simulink model "sampleModel1944_3_sub_sub_sub"  (R2023a)
settings: Solver=VariableStepAuto  StartTime=0.0  StopTime=10.0  RelTol=1e-3
libraries: hdlsllib x6, simulink x1
settings Model: Creator=user1  LastModifiedBy=user1

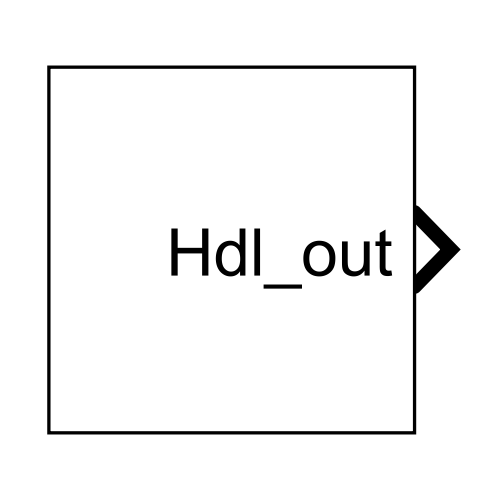
[thumbnail: Simulink's stored preview of the top-level diagram]
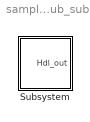
== system sampleModel1944_3_sub_sub_sub ==
  Subsystem : Subsystem

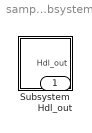
== system sampleModel1944_3_sub_sub_sub/Subsystem ==
  Subsystem : Subsystem
  Hdl_out : Outport  OutDataTypeStr=uint8

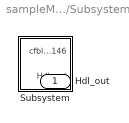
== system sampleModel1944_3_sub_sub_sub/Subsystem/Subsystem ==
  Subsystem : Subsystem
  Hdl_out : Outport  OutDataTypeStr=uint8

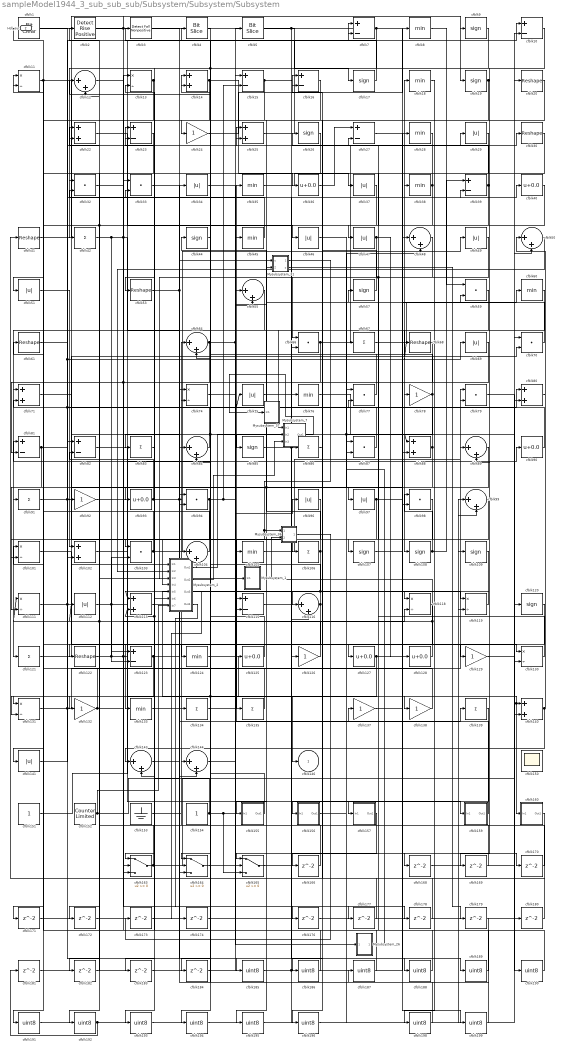
== system sampleModel1944_3_sub_sub_sub/Subsystem/Subsystem/Subsystem ==
  Mysubsystem_1 : Subsystem  TreatAsAtomicUnit=on  RTWFcnName=Mysubsystem_1
      settings: RTWFcnNameOpts=User specified  RTWFileNameOpts=Use function name
  Mysubsystem_2 : Subsystem  TreatAsAtomicUnit=on  RTWFcnName=Mysubsystem_2
      settings: RTWFcnNameOpts=User specified  RTWFileNameOpts=Use function name
  Mysubsystem_26 : Subsystem  TreatAsAtomicUnit=on  RTWFcnName=Mysubsystem_26
      settings: RTWFcnNameOpts=User specified  RTWFileNameOpts=Use function name
  Mysubsystem_31 : Subsystem  TreatAsAtomicUnit=on  RTWFcnName=Mysubsystem_31
      settings: RTWFcnNameOpts=User specified  RTWFileNameOpts=Use function name
  Mysubsystem_36 : Subsystem  TreatAsAtomicUnit=on  RTWFcnName=Mysubsystem_36
      settings: RTWFcnNameOpts=User specified  RTWFileNameOpts=Use function name
  Mysubsystem_37 : Subsystem  TreatAsAtomicUnit=on  RTWFcnName=Mysubsystem_37
      settings: RTWFcnNameOpts=User specified  RTWFileNameOpts=Use function name
  Mysubsystem_7 : Subsystem  TreatAsAtomicUnit=on  RTWFcnName=Mysubsystem_7
      settings: RTWFcnNameOpts=User specified  RTWFileNameOpts=Use function name
  cfblk1 : simulink/Logic and Bit Operations/Bit Clear  iBit=0
      settings: LibrarySourceBlock=|
      | hdlsllib/Logic and Bit
      | Operations/Bit Clear
  cfblk{7,10,15..16,23,27,39,81..82,115,123} (11 alike) : Sum  Inputs=+-  OutDataTypeStr=uint8
  cfblk{11,13,74,101,111,118..119,130..131} (9 alike) : Product  Inputs=*/  OutDataTypeStr=uint8  RndMeth=Zero  SaturateOnIntegerOverflow=on
  cfblk{14,22,25,71,80,88,102,113,140} (9 alike) : Sum  OutDataTypeStr=uint8
  cfblk{32..33,59,66,70,77,79,87,94,98,103} (11 alike) : DotProduct  OutDataTypeStr=uint8
  cfblk{12,48,50,55,64,84,89,99,104,116,143..144} (12 alike) : Sum  Inputs=|++  OutDataTypeStr=uint8
  cfblk{8,18,28,35,38,45,60,76,105,124,133} (11 alike) : MinMax  OutDataTypeStr=uint8
  cfblk{42,67,83,86,91,106,121,134..135,139} (10 alike) : Sum  Inputs=+  OutDataTypeStr=uint8
  cfblk{9,17,19,26,44,57,85,107..109,120} (11 alike) : Signum
  cfblk{29,34,37,46..47,49,51,69,75,96..97,112,141} (13 alike) : Abs  OutDataTypeStr=uint8  SaturateOnIntegerOverflow=off
  cfblk{20,30,41,53,61,68,122} (7 alike) : Reshape
  cfblk{36,40,90,93,125,127..128} (7 alike) : Bias  Bias=0.0  SaturateOnIntegerOverflow=off
  cfblk{24,78,92,126,129,132,137..138} (8 alike) : Gain  OutDataTypeStr=uint8
  cfblk150 : Scope
      settings: Floating=on
  cfblk151 : Constant  OutDataTypeStr=uint8  SampleTime=-1
  cfblk152 : hdlsllib/Sources/Counter Limited  uplimit=7  tsamp=-1
  cfblk153 : Ground
  cfblk154 : Constant  OutDataTypeStr=uint8  SampleTime=-1
  cfblk155 : Subsystem
      settings: LibrarySourceBlock=|
      | hdlsllib/Ports &
      | Subsystems/Subsystem
  cfblk156 : Subsystem
      settings: LibrarySourceBlock=|
      | hdlsllib/Ports &
      | Subsystems/Subsystem
  cfblk157 : Subsystem
      settings: LibrarySourceBlock=|
      | hdlsllib/Ports &
      | Subsystems/Subsystem
  cfblk159 : Subsystem
      settings: LibrarySourceBlock=|
      | hdlsllib/Ports &
      | Subsystems/Subsystem
  cfblk160 : Subsystem
      settings: LibrarySourceBlock=|
      | hdlsllib/Ports &
      | Subsystems/Subsystem
  cfblk163 : Switch  OutDataTypeStr=uint8  SaturateOnIntegerOverflow=off  InputSameDT=off
  cfblk164 : Switch  OutDataTypeStr=uint8  SaturateOnIntegerOverflow=off  InputSameDT=off
  cfblk165 : Switch  OutDataTypeStr=uint8  SaturateOnIntegerOverflow=off  InputSameDT=off
  cfblk{166,168..174,176..184} (17 alike) : Delay  SampleTime=1
  cfblk{185..196,198..199} (14 alike) : DataTypeConversion  OutDataTypeStr=uint8  SaturateOnIntegerOverflow=off  RndMeth=Floor
  cfblk2 : hdlsllib/Logic and Bit Operations/Detect Rise Positive  vinit=0  OutDataTypeStr=uint8
  cfblk3 : hdlsllib/Logic and Bit Operations/Detect Fall Nonpositive  vinit=0  OutDataTypeStr=uint8
  cfblk4 : hdlsllib/Logic and Bit Operations/Bit Slice  lidx=7  ridx=0
  cfblk5 : hdlsllib/Logic and Bit Operations/Bit Slice  lidx=7  ridx=0
  cfblk146 : Outport  OutDataTypeStr=uint8  VectorParamsAs1DForOutWhenUnconnected=off
  Hdl_out : Outport  Port=2  OutDataTypeStr=uint8
  wires:
  cfblk22/1 -> cfblk46/1
  cfblk8/1 -> cfblk59/1
  cfblk80/1 -> cfblk121/1
  cfblk159/1(Out1) -> cfblk35/1
  cfblk66/1 -> cfblk164/2, cfblk29/1
  cfblk36/1 -> cfblk27/1
  cfblk93/1 -> cfblk12/2, cfblk177/1, cfblk49/1
  cfblk157/1(Out1) -> cfblk165/1
  cfblk121/1 -> cfblk70/2
  cfblk41/1 -> cfblk19/1
  cfblk153/1 -> cfblk64/1
  cfblk51/1 -> cfblk102/1
  cfblk91/1 -> cfblk25/1, cfblk97/1
  cfblk5/1 -> cfblk188/1, cfblk17/1
  cfblk160/1(Out1) -> cfblk41/1
  cfblk25/1 -> cfblk7/1
  cfblk101/1 -> cfblk127/1
  cfblk119/1 -> cfblk116/1
  cfblk57/1 -> cfblk16/1
  cfblk151/1 -> cfblk10/1
  cfblk15/1 -> cfblk130/2, cfblk124/1
  cfblk16/1 -> cfblk85/1
  cfblk37/1 -> cfblk122/1
  cfblk17/1 -> cfblk3/1
  cfblk88/1 -> cfblk27/2, cfblk115/1, cfblk131/1
  cfblk60/1 -> cfblk108/1
  cfblk35/1 -> cfblk37/1
  cfblk123/1 -> cfblk104/2, cfblk131/2
  cfblk131/1 -> cfblk79/1, cfblk75/1, cfblk25/2, cfblk68/1
  cfblk112/1 -> cfblk123/2, cfblk157/1(In1)
  cfblk48/1 -> cfblk107/1, Mysubsystem_2/3(In3)
  cfblk40/1 -> cfblk155/1(In1)
  cfblk64/1 -> cfblk138/1, cfblk5/1, cfblk81/2, cfblk163/2
  cfblk107/1 -> cfblk80/1
  cfblk103/1 -> cfblk11/2, cfblk18/1
  cfblk120/1 -> cfblk133/1
  cfblk77/1 -> cfblk45/1
  cfblk87/1 -> cfblk23/1
  cfblk138/1 -> cfblk101/1
  cfblk105/1 -> cfblk89/1
  cfblk122/1 -> cfblk103/2, cfblk39/2, cfblk79/2
  cfblk128/1 -> cfblk111/1, Mysubsystem_36/2(In2)
  cfblk89/1 -> cfblk172/1, Mysubsystem_31/2(In2)
  cfblk33/1 -> cfblk185/1
  cfblk90/1 -> cfblk14/1
  cfblk81/1 -> cfblk40/1, cfblk101/2
  cfblk140/1 -> cfblk50/1, cfblk143/1
  cfblk20/1 -> cfblk24/1
  cfblk11/1 -> cfblk51/1, cfblk135/1
  cfblk53/1 -> cfblk119/1, Mysubsystem_31/1(u)
  cfblk144/1 -> cfblk137/1
  cfblk135/1 -> cfblk14/2
  cfblk82/1 -> cfblk146/1
  cfblk92/1 -> cfblk20/1
  cfblk111/1 -> cfblk7/2, cfblk34/1
  cfblk30/1 -> cfblk47/1
  cfblk130/1 -> cfblk57/1
  cfblk137/1 -> cfblk28/1
  cfblk124/1 -> cfblk140/1, cfblk160/1(In1)
  cfblk127/1 -> cfblk140/2, cfblk194/1, Mysubsystem_2/5(In5)
  cfblk94/1 -> cfblk102/2, cfblk15/2, cfblk15/1
  cfblk55/1 -> cfblk132/1
  cfblk9/1 -> cfblk42/1
  cfblk34/1 -> cfblk159/1(In1)
  cfblk106/1 -> cfblk164/3, cfblk55/1
  cfblk70/1 -> cfblk44/1
  cfblk141/1 -> cfblk82/1
  cfblk44/1 -> cfblk64/2
  cfblk125/1 -> cfblk81/1
  cfblk102/1 -> cfblk90/1
  cfblk42/1 -> cfblk123/1, cfblk125/1, cfblk104/1
  cfblk116/1 -> cfblk171/1, cfblk32/2, cfblk113/1
  cfblk69/1 -> cfblk93/1
  cfblk71/1 -> cfblk144/2
  cfblk3/1 -> cfblk94/1
  cfblk13/1 -> cfblk141/1, cfblk83/1
  cfblk7/1 -> Hdl_out/1, cfblk199/1, cfblk164/1, cfblk53/1
  cfblk83/1 -> cfblk143/2
  cfblk156/1(Out1) -> cfblk48/2
  cfblk133/1 -> cfblk84/1
  cfblk143/1 -> cfblk139/1
  cfblk104/1 -> cfblk22/1
  cfblk28/1 -> cfblk86/1
  cfblk134/1 -> cfblk55/2
  cfblk4/1 -> cfblk84/2
  cfblk2/1 -> cfblk9/1, cfblk106/1
  cfblk108/1 -> cfblk39/1, cfblk98/1
  cfblk97/1 -> cfblk111/2, cfblk59/2
  cfblk45/1 -> cfblk13/2
  cfblk23/1 -> cfblk71/1
  cfblk24/1 -> cfblk8/1
  cfblk86/1 -> cfblk156/1(In1)
  cfblk129/1 -> cfblk10/2
  cfblk29/1 -> cfblk105/1
  cfblk132/1 -> cfblk118/2, cfblk61/1
  cfblk26/1 -> cfblk92/1
  cfblk113/1 -> cfblk69/1
  cfblk39/1 -> cfblk198/1, cfblk26/1
  cfblk27/1 -> cfblk129/1
  cfblk67/1 -> cfblk60/1
  cfblk154/1 -> cfblk113/2, Mysubsystem_2/6(In6), cfblk165/3, cfblk96/1
  cfblk164/1 -> cfblk165/2
  cfblk79/1 -> cfblk120/1
  cfblk96/1 -> cfblk103/1
  cfblk85/1 -> cfblk38/1, cfblk118/1
  cfblk155/1(Out1) -> cfblk12/1
  cfblk163/1 -> cfblk50/2, cfblk82/2
  cfblk126/1 -> cfblk112/1, Mysubsystem_1/1(In1)
  cfblk14/1 -> cfblk163/3, cfblk36/1
  cfblk98/1 -> cfblk163/1
  cfblk19/1 -> cfblk186/1, cfblk89/2
  cfblk47/1 -> cfblk196/1, cfblk128/1
  cfblk115/1 -> cfblk130/1
  cfblk99/1 -> cfblk192/1
  cfblk84/1 -> cfblk11/1
  cfblk49/1 -> cfblk66/1
  cfblk78/1 -> cfblk4/1, cfblk184/1, cfblk183/1
  cfblk38/1 -> cfblk32/1, cfblk182/1, cfblk91/1
  cfblk61/1 -> cfblk30/1
  cfblk152/1 -> cfblk134/1, Mysubsystem_2/7(In7)
  cfblk46/1 -> cfblk88/1, cfblk98/2
  cfblk18/1 -> cfblk78/1
  cfblk139/1 -> cfblk166/1
  cfblk166/1 -> cfblk13/1
  cfblk165/1 -> cfblk168/1
  cfblk168/1 -> cfblk70/1
  cfblk10/1 -> cfblk169/1
  cfblk169/1 -> cfblk144/1
  cfblk75/1 -> cfblk170/1
  cfblk170/1 -> cfblk2/1
  cfblk171/1 -> cfblk119/2
  cfblk172/1 -> cfblk116/2
  cfblk173/1 -> cfblk80/2
  cfblk174/1 -> cfblk66/2
  cfblk176/1 -> cfblk48/1
  cfblk177/1 -> cfblk71/2
  cfblk32/1 -> cfblk178/1
  cfblk178/1 -> cfblk23/2
  cfblk180/1 -> cfblk16/2
  cfblk181/1 -> cfblk94/2
  cfblk182/1 -> cfblk22/2
  cfblk183/1 -> cfblk115/2
  cfblk184/1 -> cfblk88/2
  cfblk185/1 -> cfblk67/1, cfblk126/1
  cfblk186/1 -> cfblk33/1
  cfblk179/1 -> cfblk187/1
  cfblk187/1 -> cfblk33/2
  cfblk188/1 -> cfblk1/1
  cfblk1/1 -> cfblk189/1
  cfblk189/1 -> cfblk77/1
  cfblk76/1 -> cfblk190/1
  cfblk190/1 -> cfblk77/2
  cfblk68/1 -> cfblk191/1
  cfblk191/1 -> cfblk76/1
  cfblk192/1 -> cfblk180/1, cfblk181/1
  cfblk118/1 -> cfblk193/1
  cfblk193/1 -> cfblk99/1
  cfblk194/1 -> cfblk99/2
  cfblk109/1 -> cfblk195/1
  cfblk195/1 -> cfblk87/2
  cfblk196/1 -> cfblk109/1
  cfblk198/1 -> cfblk74/1
  cfblk199/1 -> cfblk74/2
  cfblk12/1 -> Mysubsystem_2/1(In1)
  cfblk50/1 -> Mysubsystem_2/2(In2)
  Mysubsystem_2/3(Out3) -> cfblk174/1
  Mysubsystem_2/4(Out4) -> cfblk176/1
  cfblk59/1 -> Mysubsystem_7/1(In1)
  Mysubsystem_2/1(Out1) -> Mysubsystem_7/2(In2)
  Mysubsystem_2/2(Out2) -> Mysubsystem_7/3(In3)
  cfblk74/1 -> Mysubsystem_26/1(In1)
  Mysubsystem_26/1(Out1) -> cfblk87/1
  Mysubsystem_31/1(Out1) -> Mysubsystem_2/4(In4), Mysubsystem_36/1(In1)
  Mysubsystem_31/2(y) -> cfblk179/1
  Mysubsystem_36/1(Out1) -> cfblk173/1
  Mysubsystem_7/1(Out1) -> Mysubsystem_37/1(In1)

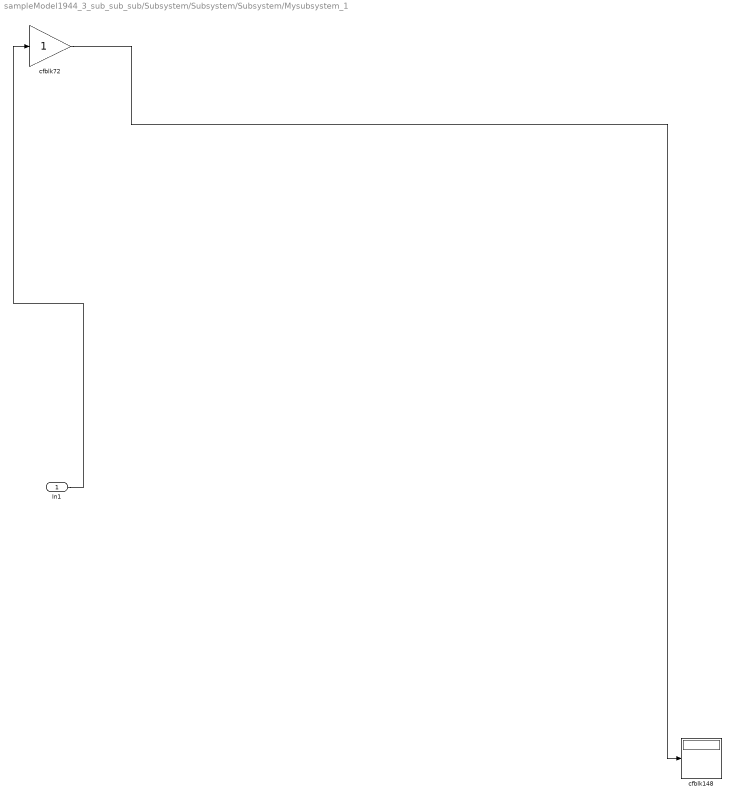
== system sampleModel1944_3_sub_sub_sub/Subsystem/Subsystem/Subsystem/Mysubsystem_1 ==
  In1 : Inport
  cfblk148 : Display
  cfblk72 : Gain
  wires:
  In1/1 -> cfblk72/1
  cfblk72/1 -> cfblk148/1

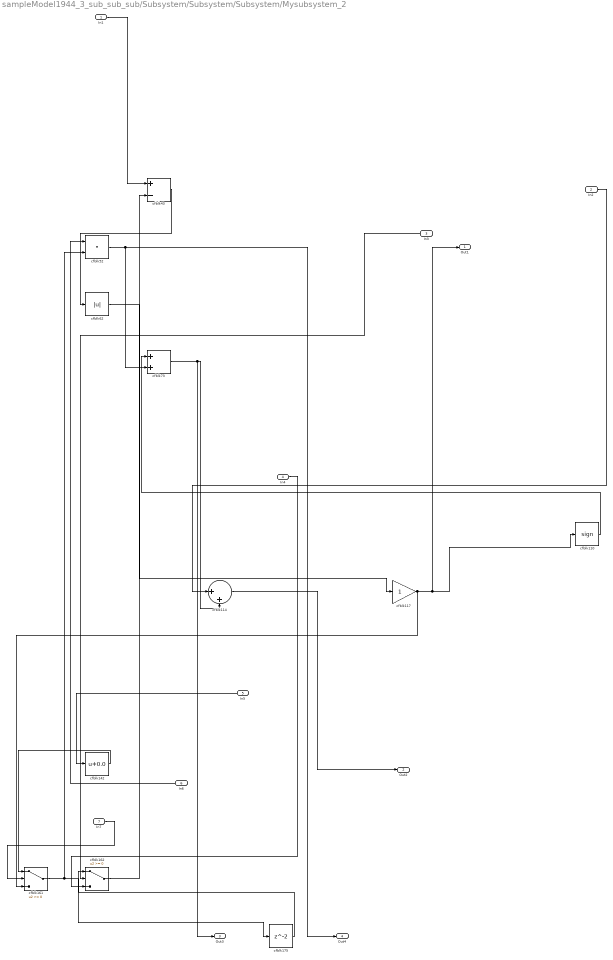
== system sampleModel1944_3_sub_sub_sub/Subsystem/Subsystem/Subsystem/Mysubsystem_2 ==
  In1 : Inport
  In2 : Inport  Port=2
  In3 : Inport  Port=3
  In4 : Inport  Port=4
  In5 : Inport  Port=5
  In6 : Inport  Port=6
  In7 : Inport  Port=7
  cfblk110 : Signum
  cfblk114 : Sum  Inputs=|++
  cfblk117 : Gain
  cfblk142 : Bias  Bias=0.0  SaturateOnIntegerOverflow=off
  cfblk161 : Switch  SaturateOnIntegerOverflow=off  InputSameDT=off
  cfblk162 : Switch  SaturateOnIntegerOverflow=off  InputSameDT=off
  cfblk175 : Delay  SampleTime=1
  cfblk43 : Sum  Inputs=+-
  cfblk52 : DotProduct  OutDataTypeStr=Inherit: Inherit via internal rule
  cfblk62 : Abs  SaturateOnIntegerOverflow=off
  cfblk73 : Sum
  Out1 : Outport
  Out2 : Outport  Port=2
  Out3 : Outport  Port=3
  Out4 : Outport  Port=4
  wires:
  In3/1 -> cfblk162/2
  In6/1 -> cfblk52/1
  In5/1 -> cfblk142/1
  In2/1 -> cfblk114/1
  cfblk114/1 -> Out2/1
  cfblk175/1 -> cfblk162/1
  cfblk162/1 -> cfblk43/2
  In4/1 -> cfblk162/3
  cfblk43/1 -> cfblk62/1
  cfblk52/1 -> cfblk73/2, Out4/1
  cfblk62/1 -> cfblk117/1
  cfblk117/1 -> cfblk161/3, cfblk110/1, Out1/1
  In1/1 -> cfblk43/1
  In7/1 -> cfblk161/2
  cfblk110/1 -> cfblk73/1
  cfblk142/1 -> cfblk161/1
  cfblk161/1 -> cfblk175/1, cfblk52/2
  cfblk73/1 -> cfblk114/2, Out3/1

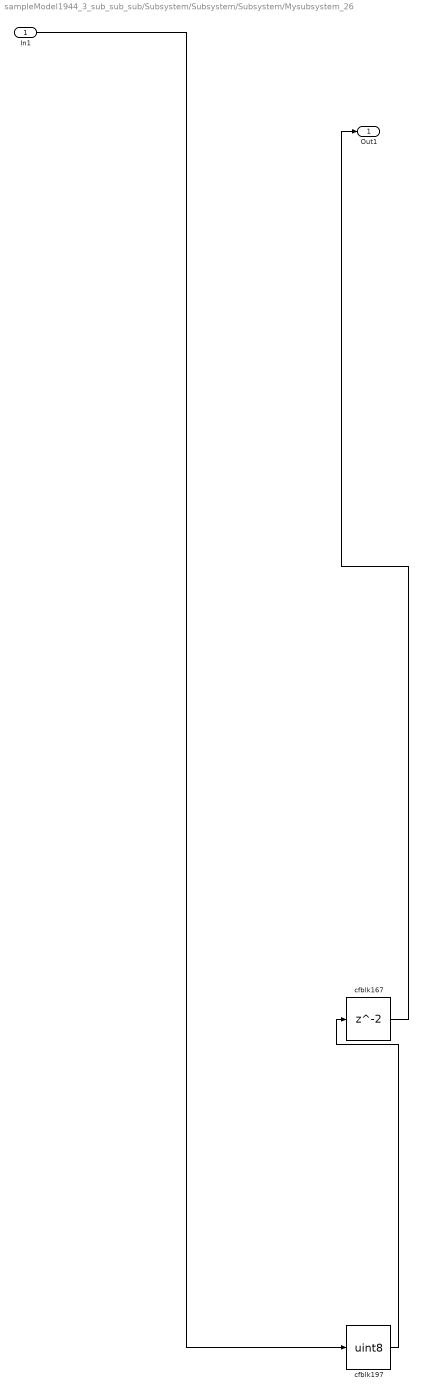
== system sampleModel1944_3_sub_sub_sub/Subsystem/Subsystem/Subsystem/Mysubsystem_26 ==
  In1 : Inport
  cfblk167 : Delay  SampleTime=1
  cfblk197 : DataTypeConversion  OutDataTypeStr=uint8  SaturateOnIntegerOverflow=off  RndMeth=Floor
  Out1 : Outport
  wires:
  In1/1 -> cfblk197/1
  cfblk167/1 -> Out1/1
  cfblk197/1 -> cfblk167/1

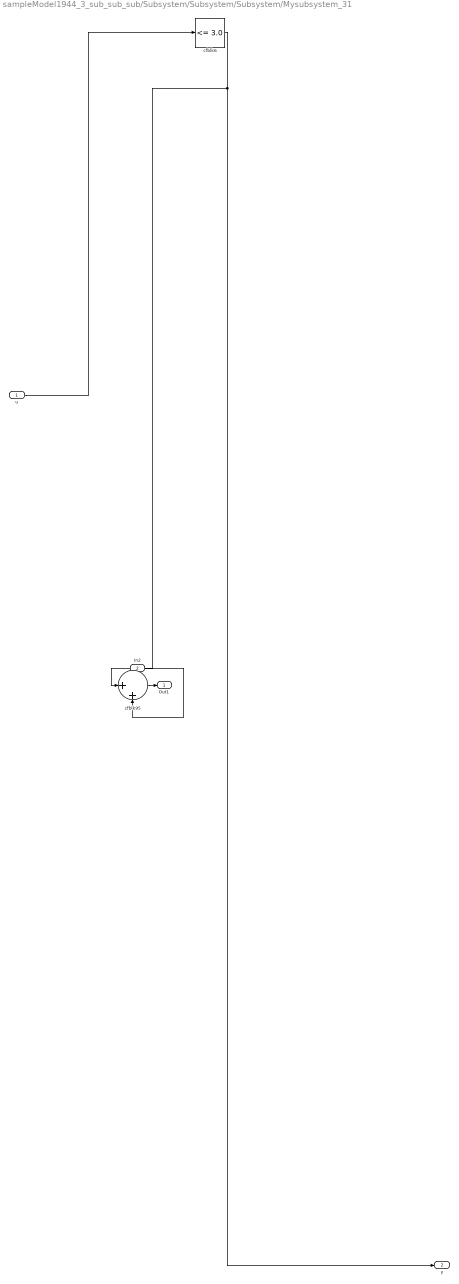
== system sampleModel1944_3_sub_sub_sub/Subsystem/Subsystem/Subsystem/Mysubsystem_31 ==
  u : Inport
  In2 : Inport  Port=2
  cfblk6 : hdlsllib/Logic and Bit Operations/Compare To Constant  relop=<=  const=3.0  OutDataTypeStr=boolean
  cfblk95 : Sum  Inputs=|++
  Out1 : Outport
  y : Outport  Port=2
  wires:
  u/1 -> cfblk6/1
  cfblk95/1 -> Out1/1
  In2/1 -> cfblk95/2
  cfblk6/1 -> cfblk95/1, y/1

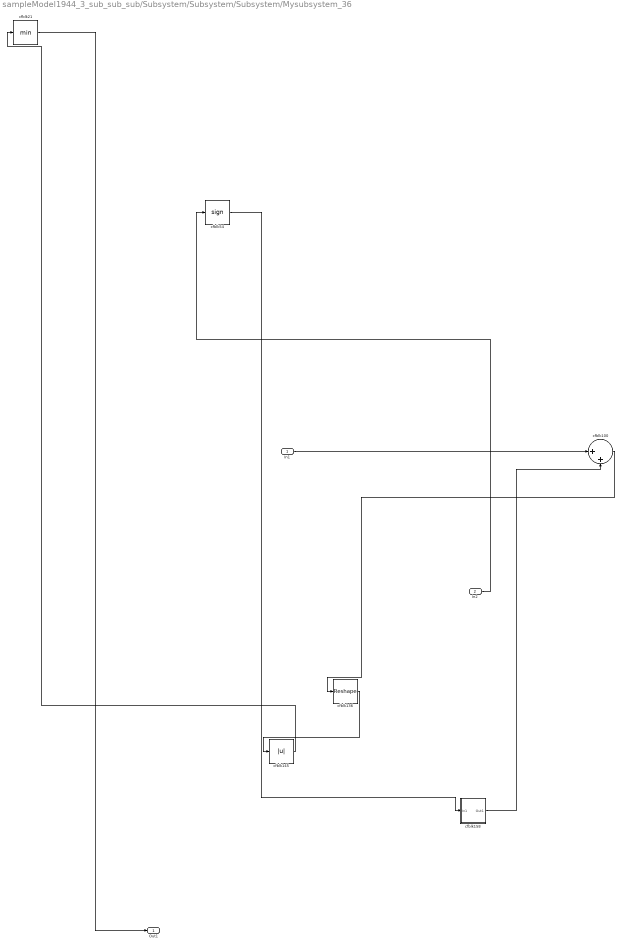
== system sampleModel1944_3_sub_sub_sub/Subsystem/Subsystem/Subsystem/Mysubsystem_36 ==
  In1 : Inport
  In2 : Inport  Port=2
  cfblk100 : Sum  Inputs=|++
  cfblk136 : Reshape
  cfblk145 : Abs  SaturateOnIntegerOverflow=off
  cfblk158 : Subsystem
      settings: LibrarySourceBlock=|
      | hdlsllib/Ports &
      | Subsystems/Subsystem
  cfblk21 : MinMax
  cfblk54 : Signum
  Out1 : Outport
  wires:
  cfblk100/1 -> cfblk136/1
  cfblk145/1 -> cfblk21/1
  In1/1 -> cfblk100/1
  In2/1 -> cfblk54/1
  cfblk54/1 -> cfblk158/1(In1)
  cfblk21/1 -> Out1/1
  cfblk158/1(Out1) -> cfblk100/2
  cfblk136/1 -> cfblk145/1

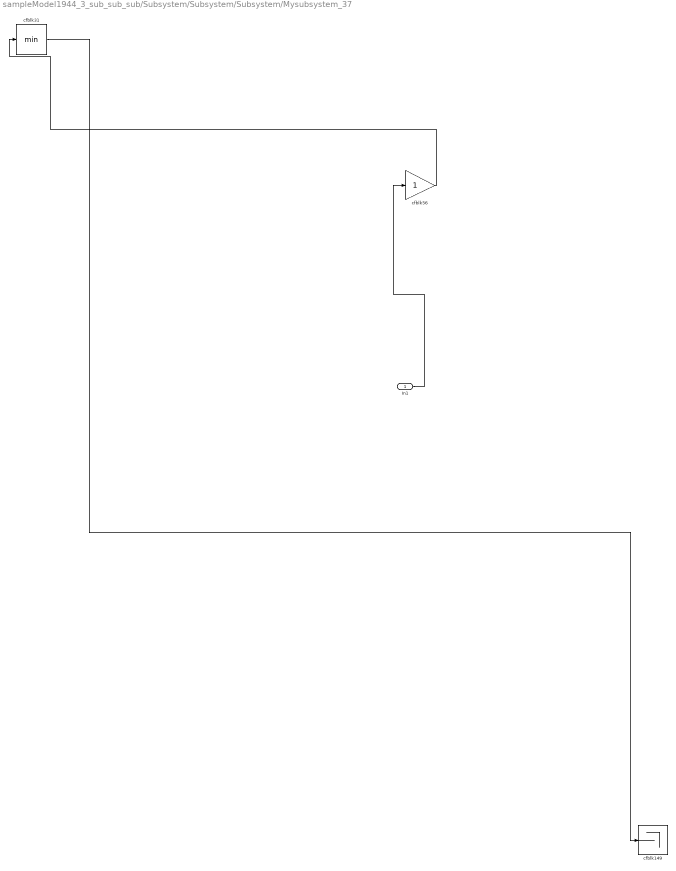
== system sampleModel1944_3_sub_sub_sub/Subsystem/Subsystem/Subsystem/Mysubsystem_37 ==
  In1 : Inport
  cfblk149 : Terminator
  cfblk31 : MinMax
  cfblk56 : Gain
  wires:
  In1/1 -> cfblk56/1
  cfblk31/1 -> cfblk149/1
  cfblk56/1 -> cfblk31/1

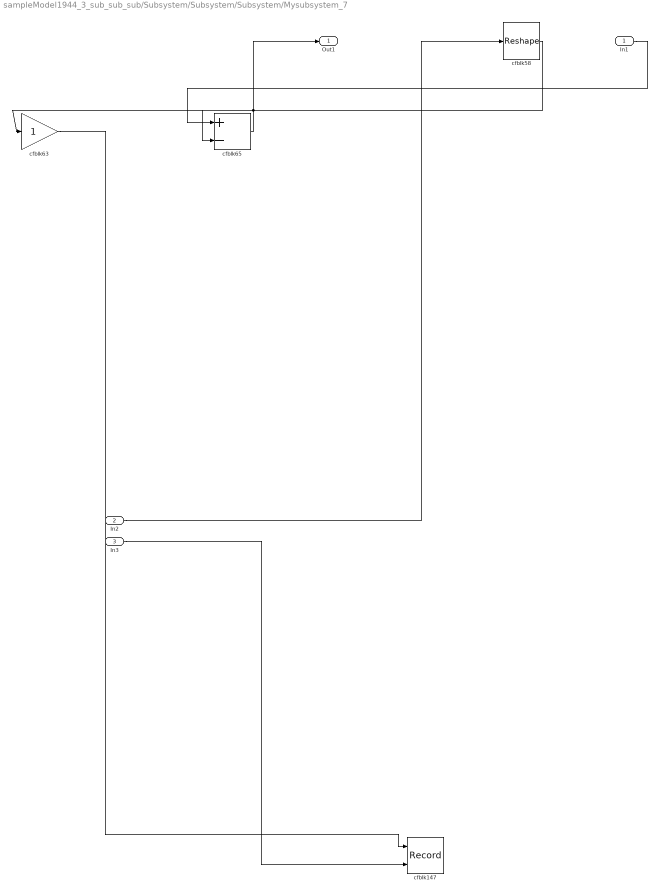
== system sampleModel1944_3_sub_sub_sub/Subsystem/Subsystem/Subsystem/Mysubsystem_7 ==
  In1 : Inport
  In2 : Inport  Port=2
  In3 : Inport  Port=3
  cfblk147 : Record  FileSettingsInternal="{\"entries\":[{\"content\":{\"excelSettings\":{\"content\":{},\"type\":\"Streamout.ExcelSettings\"}},\"type\":\"Streamout.FileSettingStorage\",\"uuid\":\"\"}],\"packageUris\":[\"http:\\/\\/schema.mathworks.com\\/mf0\\/streamout_blocks\\/R2020a\"],\"version\":\"1.0\"}"  Layout=[1 1]  SignalsInternal="{\"entries\":[{\"content\":{},\"type\":\"RecordBlkView.InputSignals\",\"uuid\":\"\"}],\"packageUris\":[\"http:\\/\\/schema.mathworks.com\\/mf0\\/streamout_blocks\\/R2020a\"],\"version\":\"1.0\"}"  VisualizationBindings="{\"xyplotplugin\":{\"info\":[{\"series\":[],\"subplotID\":1}]}}"  CompatibilityTag=XY  st=-1
  cfblk58 : Reshape
  cfblk63 : Gain
  cfblk65 : Sum  Inputs=+-
  Out1 : Outport
  wires:
  In2/1 -> cfblk58/1
  In1/1 -> cfblk65/1
  In3/1 -> cfblk147/2
  cfblk65/1 -> cfblk63/1, Out1/1
  cfblk63/1 -> cfblk147/1
  cfblk58/1 -> cfblk65/2

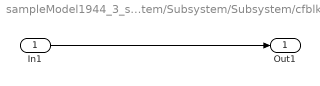
== system sampleModel1944_3_sub_sub_sub/Subsystem/Subsystem/Subsystem/cfblk155 ==
  In1 : Inport
  Out1 : Outport
  wires:
  In1/1 -> Out1/1

== system sampleModel1944_3_sub_sub_sub/Subsystem/Subsystem/Subsystem/cfblk156 ==
  In1 : Inport
  Out1 : Outport
  wires:
  In1/1 -> Out1/1

== system sampleModel1944_3_sub_sub_sub/Subsystem/Subsystem/Subsystem/cfblk157 ==
  In1 : Inport
  Out1 : Outport
  wires:
  In1/1 -> Out1/1

== system sampleModel1944_3_sub_sub_sub/Subsystem/Subsystem/Subsystem/cfblk159 ==
  In1 : Inport
  Out1 : Outport
  wires:
  In1/1 -> Out1/1

== system sampleModel1944_3_sub_sub_sub/Subsystem/Subsystem/Subsystem/cfblk160 ==
  In1 : Inport
  Out1 : Outport
  wires:
  In1/1 -> Out1/1

== system sampleModel1944_3_sub_sub_sub/Subsystem/Subsystem/Subsystem/Mysubsystem_36/cfblk158 ==
  In1 : Inport
  Out1 : Outport
  wires:
  In1/1 -> Out1/1
